simulink model "sl_groundvehicleDynamics2"  (R2024a)
settings: Solver=ode45  StartTime=0.0  StopTime=5000  RelTol=1e-5  EnableMultiTasking=on
InitFcn:
  | [waypoints,waypoint_mat,path] = wpMap;
undefined symbols (not defined in the file or in its folder): waypoint_mat, waypoints
libraries: simulink x4, mobileRoboticsLib x3, simulink_extras x2
settings Model: PacingRate=10  Creator=sriramn  LastModifiedBy=jeff
settings SolverCC: ZeroCrossAlgorithm=Adaptive  AlgebraicLoopSolver=TrustRegion
settings DataIOCC: LimitDataPoints=on  SaveFormat=Array  ReturnWorkspaceOutputs=off
settings OptimizationCC: ReuseModelBlockBuffer=off  LifeSpan=inf
settings DebuggingCC: AlgebraicLoopMsg=none  SolverPrmCheckMsg=warning  UnconnectedInputMsg=warning  UnconnectedOutputMsg=warning  UnconnectedLineMsg=warning  AllowSymbolicDim=off  SFUnexpectedBacktrackingDiag=warning  SFNoUnconditionalDefaultTransitionDiag=warning  SFExecutionAtInitializationDiag=none  ArithmeticOperatorsInVariantConditions=warning
settings ModelReferenceCC: EnableRefExpFcnMdlSchedulingChecks=on  ModelReferenceMinAlgLoopOccurrences=on  PropagateSignalLabelsOutOfModel=off
settings SFSimCC: SimUseLocalCustomCode=off  CustomCodeUndefinedFunction=UseInterfaceOnly
settings RTWCC: RTWUseLocalCustomCode=off  GPUComputeCapability=3.5
settings CodeAppCC: StateflowObjectComments=on
settings GRTTargetCC: TargetLangStandard=C89/C90 (ANSI)
settings ConfigComp: CovMetricSettings=dw  CovSaveCumulativeToWorkspaceVar=on  CovSaveSingleToWorkspaceVar=on  CovExternalEMLEnable=off  CovSFcnEnable=off
settings SimscapeCC: SimscapeNormalizeSystem=off
settings ConfigurationSet: Description=SimMechanics 2G
settings ExplorerConfigSet: InternalSimMechanicsExplorerSettings="<ExplorerConfiguration><canonicalview>planar_xy</canonicalview><AnimationSetting><BasePlaybackSpeed>1.0</BasePlaybackSpeed><PlaybackSpeedFactor>1.0</PlaybackSpeedFactor></AnimationSetting><TilePanel><TileInfo><Tiles Columns=\"1\" Count=\"1\" Rows=\"1\"><Column Left=\"2\" Weight=\"1\"/><Column Left=\"1628\"/><Row Top=\"2\" Weight=\"1\"/><Row Top=\"1072\"/><Tile Height=\"1\" Width=\"1\" X=\"0\" Y=\"0\"/></Tiles></TileInfo><SceneInfo><SceneViewer><BGColor><R>0.60000002384185791</R><G>0.60000002384185791</G><B>0.60000002384185791</B></BGColor><Camera><Position><X>0.22951840878551699</X><Y>0.32651610611526627</Y><Z>-0.27215421354393321</Z></Position><Center><X>-0.15775714411666431</X><Y>-0.15462825985839526</Y><Z>0.065702552916005602</Z></Center><Up><X>-0.56030137557930915</X><Y>0.72817587161684794</Y><Z>0.39474329445726858</Z></Up><Left>-0.21481383955700509</Left><Right>0.21481383955700509</Right><Bottom>-0.27569784609469139</Bottom><Top>0.27569784609469139</Top></Camera></SceneViewer></SceneInfo></TilePanel></ExplorerConfiguration>"

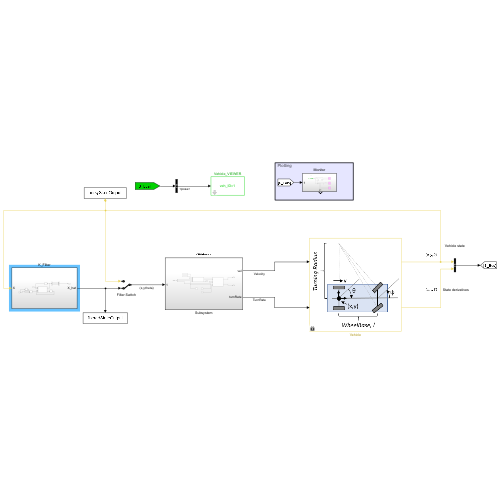
[thumbnail: Simulink's stored preview of the top-level diagram]
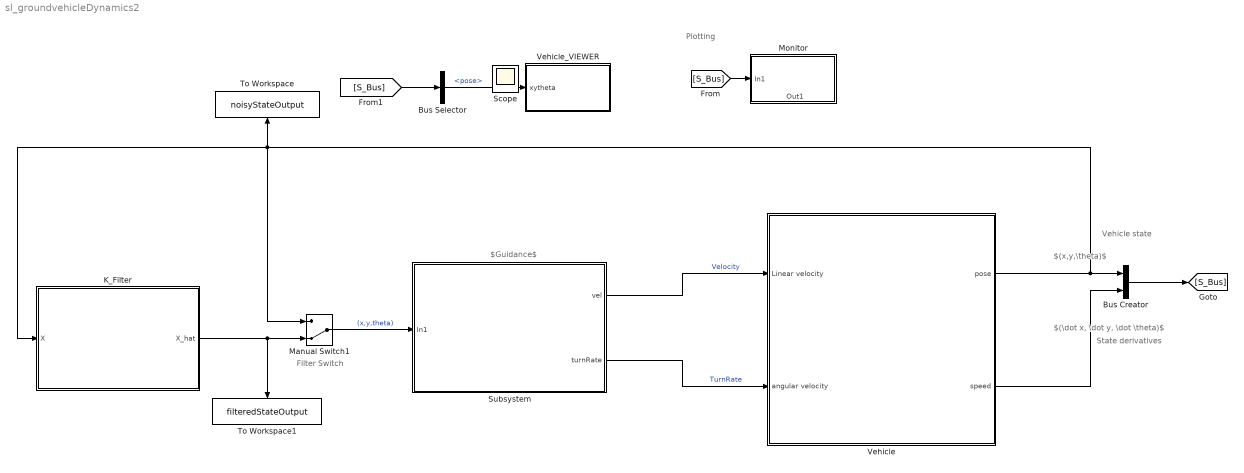
== system sl_groundvehicleDynamics2 ==
  note: State derivatives
  note: $(x,y,\theta)$
  note: $(\dot x, \dot y, \dot \theta)$
  note: Vehicle state
  note: Plotting
  note: Filter Switch
  note: $Guidance$
  Bus Creator : BusCreator  Inputs=2
  Bus Selector : BusSelector  OutputSignals=pose
  K_Filter : Subsystem
  Manual Switch1 : ManualSwitch  CurrentSetting=0
  Monitor : Subsystem
      settings: PortSchema="{\"entries\":[{\"content\":{\"sides\":[{\"content\":{\"connectorIds\":[\"In1\"]},\"type\":\"ConnectorPlacement.EquallySpacedRectSide\",\"uuid\":\"6b772a6e-a903-4be5-90e0-7e2c053b515b\"},{\"content\":{\"side\":\"RIGHT\"},\"type\":\"ConnectorPlacement.EquallySpacedRectSide\",\"uuid\":\"c575073f-211d-443d-abd5-7f48cb45a48e\"},{\"content\":{\"side\":\"TOP\"},\"type\":\"ConnectorPlacement.EquallySpacedRectSide\",\"uuid\":\"0497ffef-b6ae-4431-a12e-e3992aa83e81\"},{\"content\":{\"connectorIds\":[\"Out1\"],\"side\":\"BOTTOM\"},\"type\":\"ConnectorPlacement.EquallySpacedRectSide\",\"uuid\":\"8e6abdf5-de92-429c-ba07-6590158236d0\"}]},\"type\":\"ConnectorPlacement.EquallySpacedConnector\",\"uuid\":\"3acc5b74-a772-4792-a954-bbbdb1860183\"}],\"packageUris\":[\"http://schema.mathworks.com/mf0/Connector/R2020b\"],\"version\":\"1.0\"}"
  Subsystem : Subsystem
  To Workspace : ToWorkspace  VariableName=noisyStateOutput  SampleTime=-1
  To Workspace1 : ToWorkspace  VariableName=filteredStateOutput  SampleTime=-1
  Vehicle : Subsystem
      mask Display: image('$imagefile'); % Use "Edit Image" on toolstrip to change.
  Vehicle_VIEWER : Subsystem  mask{wp_mat=waypoint_mat, veh_ID_num=1, veh_init_xytheta=[0,0,0], Ts=0.5}
      mask prompts: wp_mat "Waypoint matrix for arena [x_col, y_col] (m)"; veh_ID_num "Vehicle ID number"; veh_init_xytheta "Initial pose [x,y,theta]"; Ts "Sample time for updating animation (secs)"
      mask TypeOptions veh_ID_num: 1 | 2 | 3 | 4
      mask DialogControl Control2 Prompt: Animate simulation of Differential Drive Robot (DDR)
      mask Display: fprintf('veh_ID=%d',veh_ID_num);
  Scope : Scope
  wires:
  [S_Bus] -> Monitor/1(In1)
  [S_Bus] -> Bus Selector/1
  Vehicle/1(pose) -> K_Filter/1(X), Manual Switch1/1, To Workspace/1, Bus Creator/1
  Bus Creator/1 -> [S_Bus]
  Bus Selector/1 -> Vehicle_VIEWER/1(xytheta)  "<pose>"
  Vehicle/2(speed) -> Bus Creator/2
  K_Filter/1(X_hat) -> Manual Switch1/2, To Workspace1/1
  Manual Switch1/1 -> Subsystem/1(In1)  "(x,y,theta)"
  Subsystem/1(vel) -> Vehicle/1(Linear velocity)  "Velocity"
  Subsystem/2(turnRate) -> Vehicle/2(angular velocity)  "TurnRate"

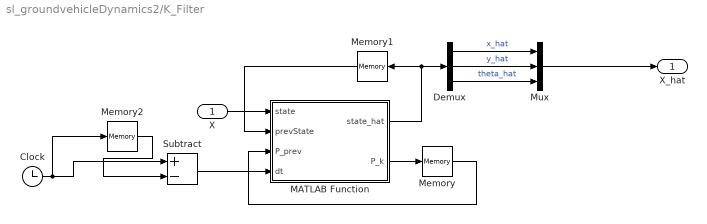
== system sl_groundvehicleDynamics2/K_Filter ==
  X : Inport
  Clock : Clock
  Demux : Demux  Outputs=3
  MATLAB Function : MATLAB Function  TreatAsAtomicUnit=on
  Memory : Memory  InheritSampleTime=on
  Memory1 : Memory  InheritSampleTime=on
  Memory2 : Memory
  Mux : Mux  Inputs=3
  Subtract : Sum  Inputs=+-
  X_hat : Outport  OutMin=3  OutMax=3
  wires:
  X/1 -> MATLAB Function/1(state)
  MATLAB Function/2(P_k) -> Memory/1
  Memory/1 -> MATLAB Function/3(P_prev)
  MATLAB Function/1(state_hat) -> Memory1/1, Demux/1
  Memory1/1 -> MATLAB Function/2(prevState)
  Subtract/1 -> MATLAB Function/4(dt)
  Clock/1 -> Subtract/1, Memory2/1
  Memory2/1 -> Subtract/2
  Demux/2 -> Mux/2  "y_hat"
  Demux/3 -> Mux/3  "theta_hat"
  Demux/1 -> Mux/1  "x_hat"
  Mux/1 -> X_hat/1

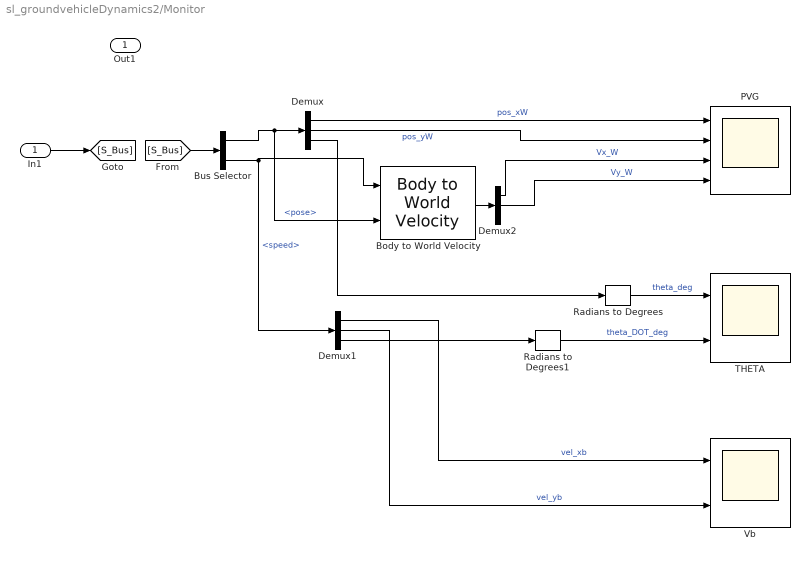
== system sl_groundvehicleDynamics2/Monitor ==
  In1 : Inport
  Body to World Velocity : mobileRoboticsLib/Utilities/Body to World Velocity
      settings: SourceProductName=Mobile Robotics Simulation Toolbox
  Bus Selector : BusSelector  OutputSignals=pose,speed
  Demux : Demux  Outputs=3
  Demux1 : Demux  Outputs=3
  Demux2 : Demux  Outputs=3
  PVG : Scope  NumInputPorts=4
  Radians to Degrees : simulink_extras/Transformations/Radians to Degrees
  Radians to Degrees1 : simulink_extras/Transformations/Radians to Degrees
  THETA : Scope  NumInputPorts=2
  Vb : Scope  NumInputPorts=2
  Out1 : Outport
  wires:
  In1/1 -> [S_Bus]
  [S_Bus] -> Bus Selector/1
  Demux/1 -> PVG/1  "pos_xW"
  Demux/2 -> PVG/2  "pos_yW"
  Radians to Degrees1/1 -> THETA/2  "theta_DOT_deg"
  Radians to Degrees/1 -> THETA/1  "theta_deg"
  Demux1/3 -> Radians to Degrees1/1
  Demux/3 -> Radians to Degrees/1
  Bus Selector/1 -> Body to World Velocity/2, Demux/1  "<pose>"
  Bus Selector/2 -> Demux1/1, Body to World Velocity/1  "<speed>"
  Body to World Velocity/1 -> Demux2/1
  Demux2/1 -> PVG/3  "Vx_W"
  Demux2/2 -> PVG/4  "Vy_W"
  Demux1/1 -> Vb/1  "vel_xb"
  Demux1/2 -> Vb/2  "vel_yb"

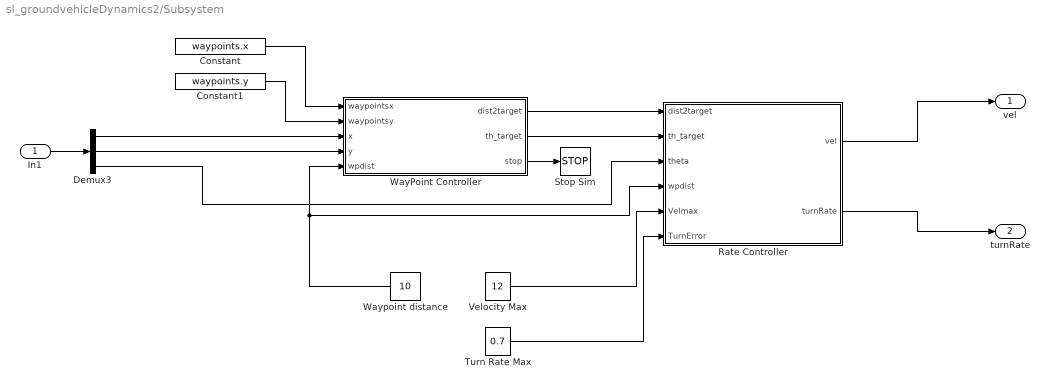
== system sl_groundvehicleDynamics2/Subsystem ==
  In1 : Inport
  Constant : Constant  Value=waypoints.x
  Constant1 : Constant  Value=waypoints.y
  Demux3 : Demux  Outputs=3
  Rate Controller : MATLAB Function  TreatAsAtomicUnit=on
  Stop Sim : Stop
  Turn Rate Max : Constant  Value=0.7
  Velocity Max : Constant  Value=12
  WayPoint Controller : MATLAB Function  TreatAsAtomicUnit=on
  Waypoint distance : Constant  Value=10
  vel : Outport
  turnRate : Outport  Port=2
  wires:
  Demux3/2 -> WayPoint Controller/4(y)
  Turn Rate Max/1 -> Rate Controller/6(TurnError)
  Demux3/1 -> WayPoint Controller/3(x)
  Waypoint distance/1 -> WayPoint Controller/5(wpdist), Rate Controller/4(wpdist)
  Constant1/1 -> WayPoint Controller/2(waypointsy)
  WayPoint Controller/1(dist2target) -> Rate Controller/1(dist2target)
  Demux3/3 -> Rate Controller/3(theta)
  Velocity Max/1 -> Rate Controller/5(Velmax)
  Constant/1 -> WayPoint Controller/1(waypointsx)
  WayPoint Controller/2(th_target) -> Rate Controller/2(th_target)
  WayPoint Controller/3(stop) -> Stop Sim/1
  In1/1 -> Demux3/1
  Rate Controller/1(vel) -> vel/1
  Rate Controller/2(turnRate) -> turnRate/1

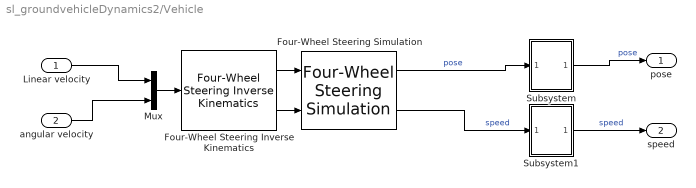
== system sl_groundvehicleDynamics2/Vehicle ==
  Linear velocity : Inport
  angular velocity : Inport  Port=2
  Four-Wheel Steering Inverse Kinematics : mobileRoboticsLib/Kinematic Models/Four-Wheel Steering/Four-Wheel Steering Inverse Kinematics  wheelRadius=0.1  frontWheelDist=0.25  rearWheelDist=0.25  ikMode=Front Steering
      settings: SourceProductName=Mobile Robotics Simulation Toolbox
  Four-Wheel Steering Simulation : mobileRoboticsLib/Kinematic Models/Four-Wheel Steering/Four-Wheel Steering Simulation  wheelRadius=0.1  frontWheelDist=0.25  rearWheelDist=0.25  initX=0  initY=0  initAngle=0  Ts=0.05
      settings: SourceProductName=Mobile Robotics Simulation Toolbox
  Mux : Mux  Inputs=2
  Subsystem : Subsystem
  Subsystem1 : Subsystem
  pose : Outport  VectorParamsAs1DForOutWhenUnconnected=off
  speed : Outport  Port=2
  wires:
  angular velocity/1 -> Mux/2
  Linear velocity/1 -> Mux/1
  Mux/1 -> Four-Wheel Steering Inverse Kinematics/1
  Four-Wheel Steering Simulation/1 -> Subsystem/1(In1)  "pose"
  Four-Wheel Steering Simulation/2 -> Subsystem1/1(In1)  "speed"
  Four-Wheel Steering Inverse Kinematics/1 -> Four-Wheel Steering Simulation/1
  Four-Wheel Steering Inverse Kinematics/2 -> Four-Wheel Steering Simulation/2
  Subsystem/1(pose) -> pose/1  "pose"
  Subsystem1/1(speed) -> speed/1  "speed"

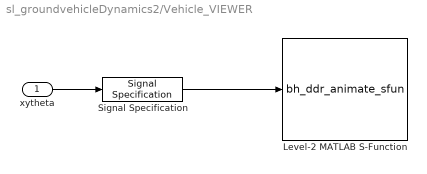
== system sl_groundvehicleDynamics2/Vehicle_VIEWER ==
  xytheta : Inport
  Level-2 MATLAB S-Function : M-S-Function  FunctionName=bh_ddr_animate_sfun  Parameters=Ts, wp_mat, veh_ID_num, veh_init_xytheta
  Signal Specification : SignalSpecification  Dimensions=3
  wires:
  xytheta/1 -> Signal Specification/1
  Signal Specification/1 -> Level-2 MATLAB S-Function/1

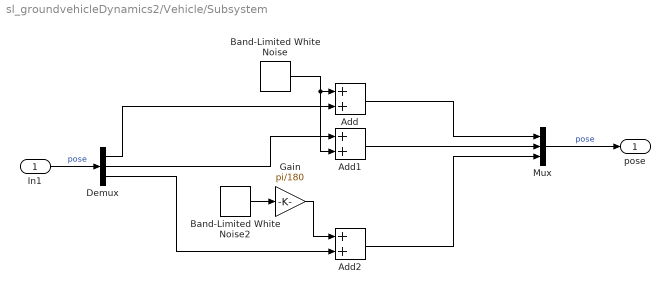
== system sl_groundvehicleDynamics2/Vehicle/Subsystem ==
  In1 : Inport
  Add : Sum
  Add1 : Sum
  Add2 : Sum
  Band-Limited White Noise : simulink/Sources/Band-Limited White Noise  Cov=[0.001]  Ts=0.1  seed=[23341]
  Band-Limited White Noise2 : simulink/Sources/Band-Limited White Noise  Cov=[0.41]  Ts=0.1  seed=[23341]
  Demux : Demux  Outputs=3
  Gain : Gain  Gain=pi/180
  Mux : Mux  Inputs=3
  pose : Outport
  wires:
  Add1/1 -> Mux/2
  Add2/1 -> Mux/3
  Demux/2 -> Add1/1
  Band-Limited White Noise2/1 -> Gain/1
  Demux/3 -> Add2/2
  Band-Limited White Noise/1 -> Add1/2, Add/1
  In1/1 -> Demux/1  "pose"
  Demux/1 -> Add/2
  Gain/1 -> Add2/1
  Mux/1 -> pose/1  "pose"
  Add/1 -> Mux/1

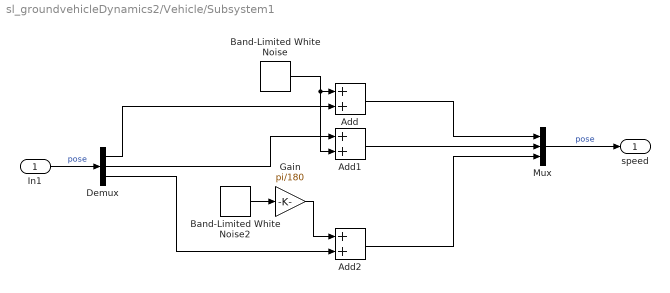
== system sl_groundvehicleDynamics2/Vehicle/Subsystem1 ==
  In1 : Inport
  Add : Sum
  Add1 : Sum
  Add2 : Sum
  Band-Limited White Noise : simulink/Sources/Band-Limited White Noise  Cov=[0.001]  Ts=0.1  seed=[23341]
  Band-Limited White Noise2 : simulink/Sources/Band-Limited White Noise  Cov=[0.41]  Ts=0.1  seed=[23341]
  Demux : Demux  Outputs=3
  Gain : Gain  Gain=pi/180
  Mux : Mux  Inputs=3
  speed : Outport
  wires:
  Add1/1 -> Mux/2
  Add2/1 -> Mux/3
  Demux/2 -> Add1/1
  Band-Limited White Noise2/1 -> Gain/1
  Demux/3 -> Add2/2
  Band-Limited White Noise/1 -> Add1/2, Add/1
  In1/1 -> Demux/1  "pose"
  Demux/1 -> Add/2
  Gain/1 -> Add2/1
  Mux/1 -> speed/1  "pose"
  Add/1 -> Mux/1

== matlab function sl_groundvehicleDynamics2/Subsystem/WayPoint Controller ==
  data: waypointsx input; waypointsy input; x input; dist2target output; y input; th_target output; stop output; wpdist input
function [dist2target,th_target,stop] = fcn(waypointsx,waypointsy,x,y,wpdist)

persistent WpCounter;
if isempty(WpCounter)
    WpCounter = 1; %% next waypoint
end

persistent Wpprev;
if isempty(Wpprev)
    Wpprev = WpCounter-1; %% waypoint ur currently at
end

if(Wpprev == 0)
    Next_wp = [waypointsx(WpCounter),waypointsy(WpCounter)];
    Prev_wp = [0,0];
 else
     Next_wp = [waypointsx(WpCounter),waypointsy(WpCounter)];
     Prev_wp = [waypointsx(Wpprev),waypointsy(Wpprev)];
     %Prev_wp = [0,0];
 end

dist2target = sqrt((Next_wp(2)-y)^2+(Next_wp(1)-x)^2);
distwp2wp = sqrt((Next_wp(2)-Prev_wp(2))^2+(Next_wp(1)-Prev_wp(1))^2);
dist2Last = sqrt((Prev_wp(2)-y)^2+(Prev_wp(1)-x)^2);
unitvec = [Next_wp(1)-Prev_wp(1),Next_wp(2)-Prev_wp(2)]/distwp2wp;

sigma = RVWP_track;
targetrel = (dist2Last+sigma)*unitvec;
target = [targetrel(1)+Prev_wp(1),targetrel(2)+Prev_wp(2)];
th_target = atan2(target(2)-y,target(1)-x);

if(dist2target < wpdist && WpCounter < 10)  
    Wpprev = WpCounter;
    WpCounter = WpCounter+1;
end

Last_wp = [waypointsx(10),waypointsy(10)];
dist2Last = sqrt((Last_wp(2)-y)^2+(Last_wp(1)-x)^2);

if(dist2Last < 1)   
    stop = 1;
else     
    stop = 0;
end

== matlab function sl_groundvehicleDynamics2/K_Filter/MATLAB Function ==
  data: state input; state_hat output; prevState input; P_prev input; P_k output; dt input
function [state_hat, P_k]= fcn(state, prevState, P_prev, dt)
%% Setup Persistent Values
persistent is_first_entry;
persistent count;

if isempty(count)
    count = 0;
end

if isempty(is_first_entry)
    is_first_entry = true;
end

%% Setup & Initial State Values
x_0 = zeros(1, 6)';
P_k = zeros(6, 6);
state_hat = state;

if ~is_first_entry
    state_hat = prevState;
    P_k = P_prev;
end


% Define the noise variance
sigma_x = 0.1;
sigma_y = 0.1;
sigma_theta = deg2rad(2); % 2 Deg in Rad

simga_x_dot = 0;
sigma_y_dot = 0;
sigma_theta_dot = 0; % RoC Degrees

R = 1.5; % Filter Gain

A = [ ...
   1, 0, 0, dt, 0, 0; ...
   0, 1, 0, 0, dt, 0; ...
   0, 0, 1, 0, 0, dt; ...
   0, 0, 0, 1, 0, 0; ...
   0, 0, 0, 0, 1, 0; ...
   0, 0, 0, 0, 0, 1 ...
  ];

H = [ ...
   1, 0, 0, 0, 0, 0; ...
   0, 1, 0, 0, 0, 0; ...
   0, 0, 1, 0, 0, 0 ...
  ];

Q = diag([sigma_x, sigma_y, sigma_theta, simga_x_dot, sigma_y_dot, sigma_theta_dot]);

R = R * eye(3);

if (is_first_entry) 
    x_kh = x_0;
    P_k = 1000 * eye(6);
else 
    x_kh = x_0;
    x_kh(1:3) = prevState;
end

%% Time Update
x_khm = A * x_kh;
P_km = A * P_k * A' + Q;

%% Measurement Update
K_k = (P_km * H') / (H * P_km * H' + R);
x_kh = x_khm + K_k * (state - H * x_khm);
P_k = (eye(6) - K_k * H) * P_km;
x_k_hat = x_kh;

% Increment internal counters
if (is_first_entry)
    count = 0;
    is_first_entry = false;
end

count = count + 1;

for i=1:3
  state_hat(i) = x_k_hat(i);
end

== matlab function sl_groundvehicleDynamics2/Subsystem/Rate Controller ==
  data: dist2target input; th_target input; theta input; wpdist input; Velmax input; TurnError input; vel output; turnRate output
function [vel,turnRate]= fcn(dist2target,th_target,theta,wpdist,Velmax,TurnError)

%% --- Control Shit ------ 
error = angdiff(theta,th_target);
K_theta = TurnError;
omega = K_theta * error;  % proportional control  - omega is the command
turnRate = omega;

persistent velocity;
if isempty(velocity)
    velocity = 0;
end
if(dist2target > wpdist)
    velocity = velocity+0.01;
    if(velocity > Velmax)
        velocity = Velmax;
    end
else
    velocity = velocity-0.01;
    if(velocity < Velmax)
        velocity = Velmax; 
    end
end
vel = velocity;
